simulink model "week2_problem3"  (R2020b)
settings: Solver=VariableStepAuto  StartTime=0.0  StopTime=10.0  RelTol=1e-3
settings Model: Creator=omkar  LastModifiedBy=omkar

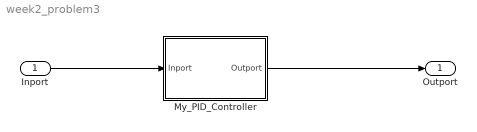
== system week2_problem3 ==
  Inport : Inport
  My_PID_Controller : Subsystem  mask{Kp=0, Ki=0, Kd=0}
      mask Display: disp('P.I.D Controller')
  Outport : Outport
  wires:
  Inport/1 -> My_PID_Controller/1(Inport)
  My_PID_Controller/1(Outport) -> Outport/1

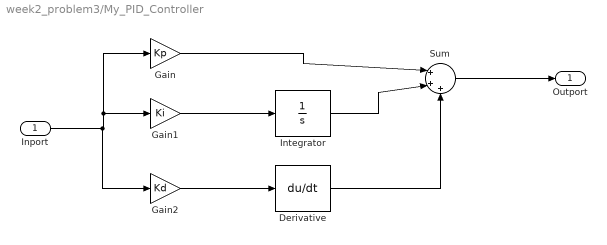
== system week2_problem3/My_PID_Controller ==
  Inport : Inport
  Derivative : Derivative
  Gain : Gain  Gain=Kp
  Gain1 : Gain  Gain=Ki
  Gain2 : Gain  Gain=Kd
  Integrator : Integrator
  Sum : Sum  Inputs=|+++
  Outport : Outport
  wires:
  Sum/1 -> Outport/1
  Gain2/1 -> Derivative/1
  Gain/1 -> Sum/1
  Derivative/1 -> Sum/3
  Gain1/1 -> Integrator/1
  Integrator/1 -> Sum/2
  Inport/1 -> Gain2/1, Gain1/1, Gain/1
